simulink model "Sistemas_Lineares"  (R2021b)
settings: Solver=VariableStepAuto  StartTime=0.0  StopTime=20  RelTol=1e-3
settings Model: Creator=gusta  LastModifiedBy=gusta

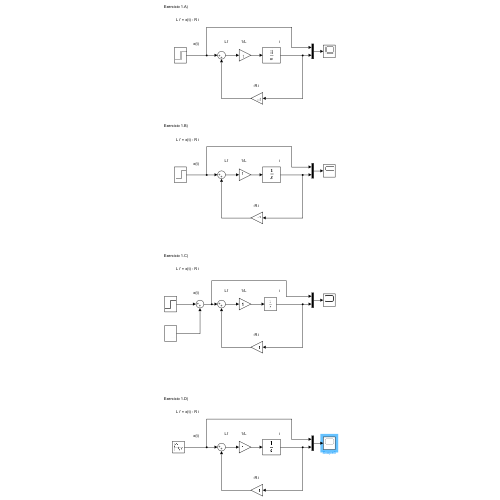
[thumbnail: Simulink's stored preview of the top-level diagram]
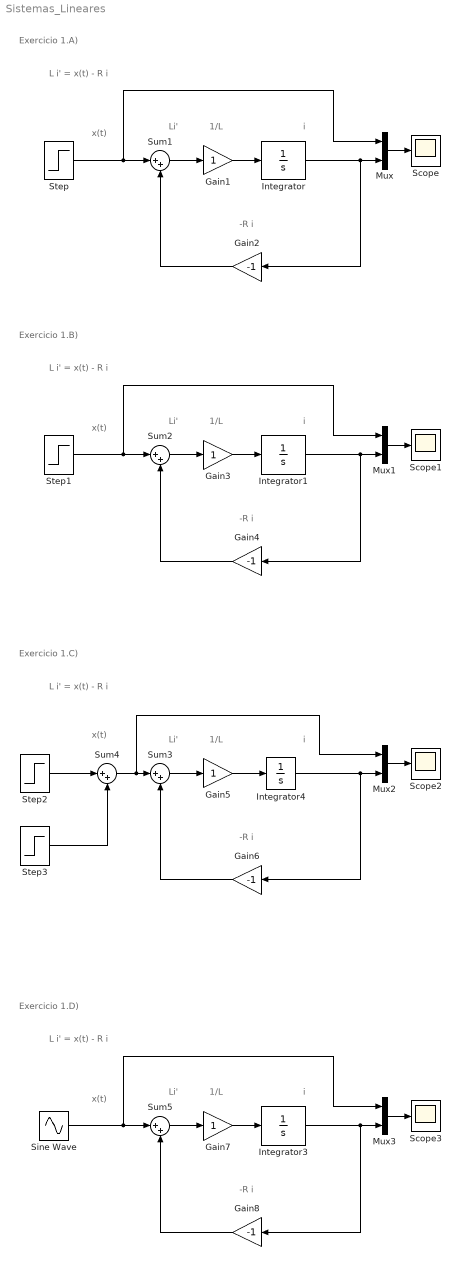
== system Sistemas_Lineares ==
  note: Exercicio 1.A)
  note: L i' = x(t) - R i
  note: Li'
  note: 1/L
  note: -R i
  note: i
  note: x(t)
  note: 1/L
  note: Exercicio 1.B)
  note: x(t)
  note: i
  note: Li'
  note: L i' = x(t) - R i
  note: -R i
  note: i
  note: x(t)
  note: Exercicio 1.C)
  note: Li'
  note: L i' = x(t) - R i
  note: -R i
  note: 1/L
  note: i
  note: x(t)
  note: Exercicio 1.D)
  note: Li'
  note: L i' = x(t) - R i
  note: -R i
  note: 1/L
  Gain{1,3,5,7} (4 alike) : Gain
  Gain{2,4,6,8} (4 alike) : Gain  Gain=-1
  Integrator{,1,3..4} (4 alike) : Integrator  InitialCondition=2
  Mux{,1..3} (4 alike) : Mux  Inputs=2
  Scope{,1..3} (4 alike) : Scope
  Sine Wave : Sin  SampleTime=0
  Step : Step  Time=0  After=0  SampleTime=0
  Step1 : Step  Time=0  SampleTime=0
  Step2 : Step  Time=0  SampleTime=0
  Step3 : Step  After=-1  SampleTime=0
  Sum{1..5} (5 alike) : Sum  Inputs=|++
  wires:
  Gain1/1 -> Integrator/1
  Sum1/1 -> Gain1/1
  Integrator/1 -> Mux/2, Gain2/1
  Gain2/1 -> Sum1/2
  Mux/1 -> Scope/1
  Step/1 -> Mux/1, Sum1/1
  Mux1/1 -> Scope1/1
  Sum2/1 -> Gain3/1
  Integrator1/1 -> Mux1/2, Gain4/1
  Gain4/1 -> Sum2/2
  Step1/1 -> Mux1/1, Sum2/1
  Gain3/1 -> Integrator1/1
  Integrator4/1 -> Gain6/1, Mux2/2
  Gain6/1 -> Sum3/2
  Mux2/1 -> Scope2/1
  Sum3/1 -> Gain5/1
  Step2/1 -> Sum4/1
  Step3/1 -> Sum4/2
  Sum4/1 -> Mux2/1, Sum3/1
  Integrator3/1 -> Mux3/2, Gain8/1
  Gain7/1 -> Integrator3/1
  Gain8/1 -> Sum5/2
  Sine Wave/1 -> Mux3/1, Sum5/1
  Mux3/1 -> Scope3/1
  Sum5/1 -> Gain7/1
  Gain5/1 -> Integrator4/1
